simulink model "Pulse_Generator"  (Simulink 7.5)
settings: Solver=ode45  StartTime=0.0  StopTime=10.0  RelTol=1e-3
settings Model: Creator=lm  LastModifiedBy=lm

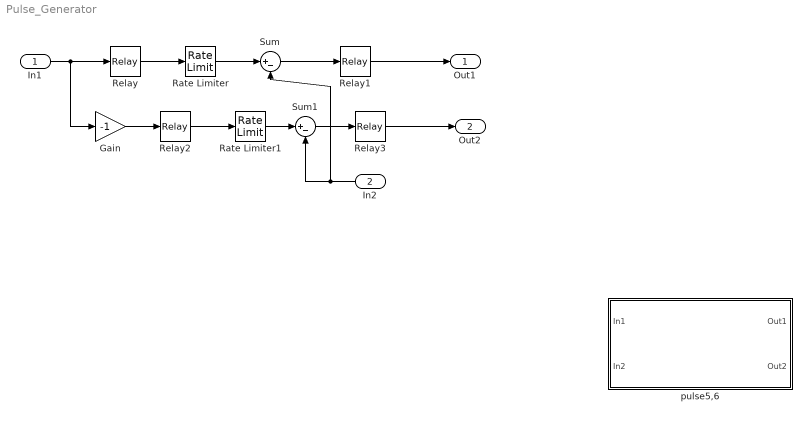
== system Pulse_Generator ==
  In1 : Inport  OutDataType=fixdt(1, 16)  OutScaling=2^0
  In2 : Inport  Port=2  OutDataType=fixdt(1, 16)  OutScaling=2^0
  Gain : Gain  Gain=-1  ParameterDataType=fixdt(1, 16)  ParameterScaling=2^0  OutDataType=fixdt(1, 16)  OutScaling=2^0
  Rate Limiter : RateLimiter  RisingSlewLimit=1000  FallingSlewLimit=-1e8  SampleTimeMode=inherited
  Rate Limiter1 : RateLimiter  RisingSlewLimit=1000  FallingSlewLimit=-1e9  SampleTimeMode=inherited
  Relay : Relay  OnOutputValue=10  OutDataType=fixdt(1, 16)  OutScaling=2^0
  Relay1 : Relay  OutDataType=fixdt(1, 16)  OutScaling=2^0
  Relay2 : Relay  OnOutputValue=10  OutDataType=fixdt(1, 16)  OutScaling=2^0
  Relay3 : Relay  OutDataType=fixdt(1, 16)  OutScaling=2^0
  Sum : Sum  Inputs=|+-  OutDataType=fixdt(1, 16)  OutScaling=2^0
  Sum1 : Sum  Inputs=|+-  OutDataType=fixdt(1, 16)  OutScaling=2^0
  pulse5,6 : Subsystem
  Out1 : Outport  OutDataType=fixdt(1, 16)  OutScaling=2^0
  Out2 : Outport  Port=2  OutDataType=fixdt(1, 16)  OutScaling=2^0
  wires:
  Rate Limiter/1 -> Sum/1
  Relay/1 -> Rate Limiter/1
  Relay3/1 -> Out2/1
  Sum1/1 -> Relay3/1
  In2/1 -> Sum/2, Sum1/2
  Rate Limiter1/1 -> Sum1/1
  Relay2/1 -> Rate Limiter1/1
  Gain/1 -> Relay2/1
  In1/1 -> Gain/1, Relay/1
  Sum/1 -> Relay1/1
  Relay1/1 -> Out1/1

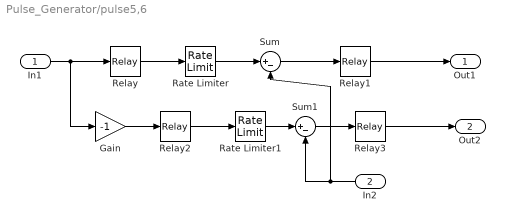
== system Pulse_Generator/pulse5,6 ==
  In1 : Inport  OutDataType=fixdt(1, 16)  OutScaling=2^0
  In2 : Inport  Port=2  OutDataType=fixdt(1, 16)  OutScaling=2^0
  Gain : Gain  Gain=-1  ParameterDataType=fixdt(1, 16)  ParameterScaling=2^0  OutDataType=fixdt(1, 16)  OutScaling=2^0
  Rate Limiter : RateLimiter  RisingSlewLimit=1000  FallingSlewLimit=-1e8  SampleTimeMode=inherited
  Rate Limiter1 : RateLimiter  RisingSlewLimit=1000  FallingSlewLimit=-1e9  SampleTimeMode=inherited
  Relay : Relay  OnOutputValue=10  OutDataType=fixdt(1, 16)  OutScaling=2^0
  Relay1 : Relay  OutDataType=fixdt(1, 16)  OutScaling=2^0
  Relay2 : Relay  OnOutputValue=10  OutDataType=fixdt(1, 16)  OutScaling=2^0
  Relay3 : Relay  OutDataType=fixdt(1, 16)  OutScaling=2^0
  Sum : Sum  Inputs=|+-  OutDataType=fixdt(1, 16)  OutScaling=2^0
  Sum1 : Sum  Inputs=|+-  OutDataType=fixdt(1, 16)  OutScaling=2^0
  Out1 : Outport  OutDataType=fixdt(1, 16)  OutScaling=2^0
  Out2 : Outport  Port=2  OutDataType=fixdt(1, 16)  OutScaling=2^0
  wires:
  Rate Limiter/1 -> Sum/1
  Relay/1 -> Rate Limiter/1
  Relay3/1 -> Out2/1
  Sum1/1 -> Relay3/1
  In2/1 -> Sum/2, Sum1/2
  Rate Limiter1/1 -> Sum1/1
  Relay2/1 -> Rate Limiter1/1
  Gain/1 -> Relay2/1
  In1/1 -> Gain/1, Relay/1
  Sum/1 -> Relay1/1
  Relay1/1 -> Out1/1
